simulink model "UAV_altitude"  (R2024b)
settings: Solver=ode4  StartTime=0.0  StopTime=simulation_time  FixedStep=sample_time  RelTol=1e-3
values from neighbouring files (symbols this model uses):
  k1 = 1    [Step3_UAV_altitude.m]
  k2 = 2    [Step3_UAV_altitude.m]
undefined symbols (not defined in the file or in its folder): i
libraries: uavutilslib x1
settings Model: Creator=zhes  LastModifiedBy=zhes

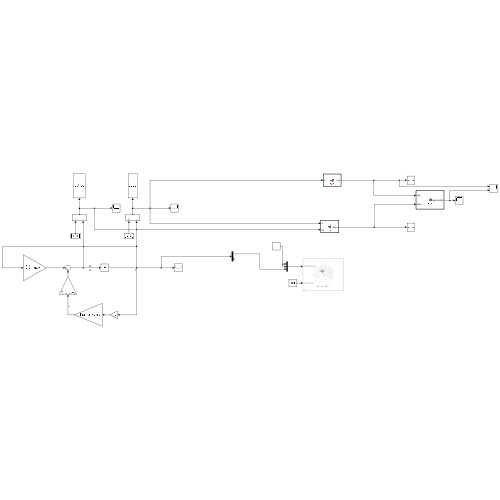
[thumbnail: Simulink's stored preview of the top-level diagram]
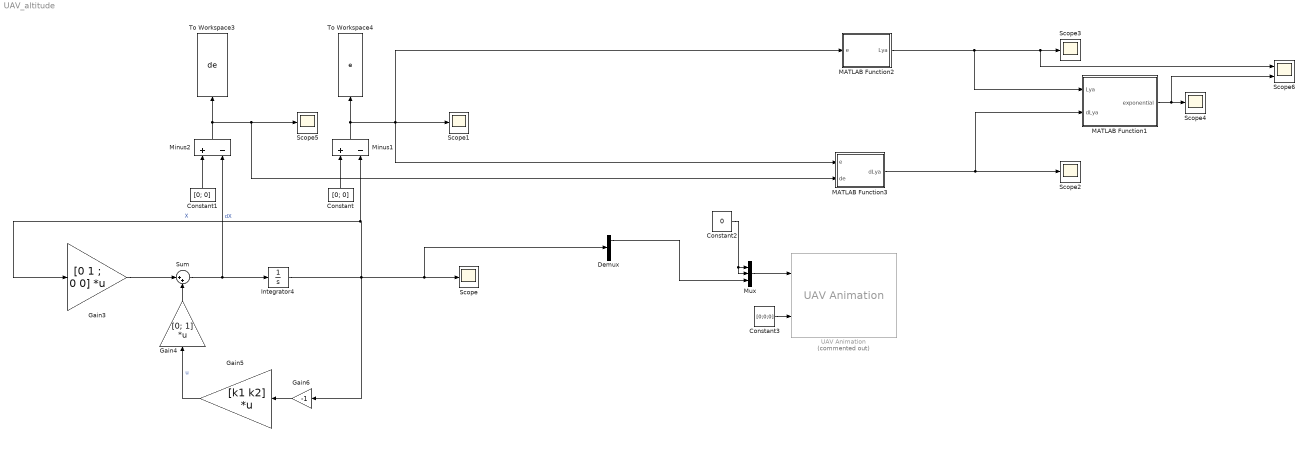
== system UAV_altitude ==
  Constant : Constant  Value=[0; 0]
  Constant1 : Constant  Value=[0; 0]
  Constant2 : Constant  Value=0
  Constant3 : Constant  Value=[0;0;0]
  Demux : Demux  Outputs=2
  Gain3 : Gain  Gain="[0  1 ; 0  0]"  Multiplication=Matrix(K*u) (u vector)
  Gain4 : Gain  Gain=[0; 1]  Multiplication=Matrix(K*u) (u vector)
  Gain5 : Gain  Gain="[k1  k2]"  Multiplication=Matrix(K*u) (u vector)
  Gain6 : Gain  Gain=-1
  Integrator4 : Integrator  InitialCondition=[0.8/i; 0.5/i]
  MATLAB Function1 : MATLAB Function  TreatAsAtomicUnit=on
  MATLAB Function2 : MATLAB Function  TreatAsAtomicUnit=on
  MATLAB Function3 : MATLAB Function  TreatAsAtomicUnit=on
  Minus1 : Sum  Inputs=+-
  Minus2 : Sum  Inputs=+-
  Mux : Mux  Inputs=3
  Scope{,1..5} (6 alike) : Scope
  Scope6 : Scope  NumInputPorts=2
  Sum : Sum  Inputs=|++
  To Workspace3 : ToWorkspace  VariableName=de  SaveFormat=Structure With Time  SampleTime=-1
  To Workspace4 : ToWorkspace  VariableName=e  SaveFormat=Structure With Time  SampleTime=-1
  UAV Animation : uavutilslib/UAV Animation  Commented=on  NumUAV=1  DynamicUAVConfig=off  UAVType=Multirotor  UAVSize=1  UAVColor=[1 0 0]  UAVTrajectoryAlpha=1  InertialZDirection=Up  RotationFormat=Euler ZYX  DrawMarkers=off  SampleTime=-1
  wires:
  Integrator4/1 -> Demux/1, Scope/1, Gain3/1, Minus1/2, Gain6/1  "X"
  Gain3/1 -> Sum/1
  Gain4/1 -> Sum/2
  Gain5/1 -> Gain4/1  "u"
  Gain6/1 -> Gain5/1
  Constant/1 -> Minus1/1
  Sum/1 -> Minus2/2, Integrator4/1  "dX"
  Constant1/1 -> Minus2/1
  Minus1/1 -> To Workspace4/1, MATLAB Function3/1(e), MATLAB Function2/1(e), Scope1/1
  Minus2/1 -> MATLAB Function3/2(de), Scope5/1, To Workspace3/1
  MATLAB Function1/1(exponential) -> Scope6/2, Scope4/1
  MATLAB Function2/1(Lya) -> MATLAB Function1/1(Lya), Scope6/1, Scope3/1
  MATLAB Function3/1(dLya) -> MATLAB Function1/2(dLya), Scope2/1
  Mux/1 -> UAV Animation/1
  Demux/1 -> Mux/3
  Constant2/1 -> Mux/2, Mux/1
  Constant3/1 -> UAV Animation/2

== matlab function UAV_altitude/MATLAB Function2 ==
  data: e input; Lya output
function Lya = fcn(e)

A = [ 1.103377375919055   0.986454393516947
   0.986454393516947   1.106107676588471 ]; % lambda = 1

Lya = e.' * A * e;

== matlab function UAV_altitude/MATLAB Function3 ==
  data: e input; dLya output; de input
function dLya = fcn(e, de)

de1 = e(1);
de2 = e(2);

dde1 = de(1);
dde2 = de(2);


A = [ 1.103377375919055   0.986454393516947
   0.986454393516947   1.106107676588471 ]; % lambda = 1

dLya = de' * A * e + e' * A * de;

== matlab function UAV_altitude/MATLAB Function1 ==
  data: Lya input; exponential output; dLya input
function exponential = fcn(Lya, dLya)

lambda = 1;

exponential = dLya + lambda * Lya;
